simulink model "perceptron"  (R2021a)
settings: Solver=VariableStepAuto  StartTime=0.0  StopTime=10.0  RelTol=1e-3
settings Model: Creator=User  LastModifiedBy=User

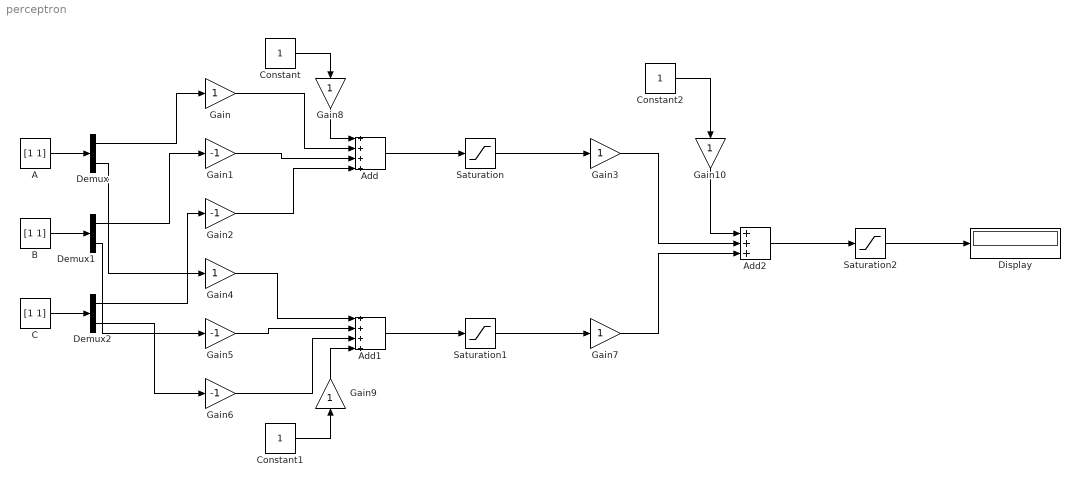
== system perceptron ==
  A : Constant  Value=[1 1]
  Add : Sum  Inputs=++++
  Add1 : Sum  Inputs=++++
  Add2 : Sum  Inputs=+++
  B : Constant  Value=[1 1]
  C : Constant  Value=[1 1]
  Constant : Constant
  Constant1 : Constant
  Constant2 : Constant
  Demux : Demux  Outputs=2
  Demux1 : Demux  Outputs=2
  Demux2 : Demux  Outputs=2
  Display : Display
  Gain{,3..4,7..10} (7 alike) : Gain
  Gain{1..2,5..6} (4 alike) : Gain  Gain=-1
  Saturation : Saturate  UpperLimit=1  LowerLimit=0
  Saturation1 : Saturate  UpperLimit=1  LowerLimit=0
  Saturation2 : Saturate  UpperLimit=1  LowerLimit=0
  wires:
  A/1 -> Demux/1
  B/1 -> Demux1/1
  Gain/1 -> Add/2
  Gain1/1 -> Add/3
  Add/1 -> Saturation/1
  Saturation/1 -> Gain3/1
  Gain2/1 -> Add/4
  C/1 -> Demux2/1
  Saturation1/1 -> Gain7/1
  Gain6/1 -> Add1/3
  Add1/1 -> Saturation1/1
  Gain4/1 -> Add1/1
  Gain5/1 -> Add1/2
  Gain3/1 -> Add2/2
  Gain7/1 -> Add2/3
  Add2/1 -> Saturation2/1
  Saturation2/1 -> Display/1
  Demux/1 -> Gain/1
  Demux/2 -> Gain4/1
  Demux1/1 -> Gain1/1
  Demux1/2 -> Gain5/1
  Demux2/1 -> Gain2/1
  Demux2/2 -> Gain6/1
  Constant/1 -> Gain8/1
  Gain8/1 -> Add/1
  Constant1/1 -> Gain9/1
  Gain9/1 -> Add1/4
  Constant2/1 -> Gain10/1
  Gain10/1 -> Add2/1
